simulink model "ModelWithPV"  (R2018a)
settings: Solver=FixedStepAuto  StartTime=0.0  StopTime=1.66  FixedStep=0.01  RelTol=1e-3
PreLoadFcn:
  | myparameterswithpv;
InitFcn:
  | myparameterswithpv;
StopFcn:
  | %datawriter;
values from neighbouring files (symbols this model uses):
  max_p = max(ut_price_i)    [myparametersnopv.m]    (also in myparameterswithpv.m)
libraries: fuzblock x1
settings Model: Creator=timothy  LastModifiedBy=timothy

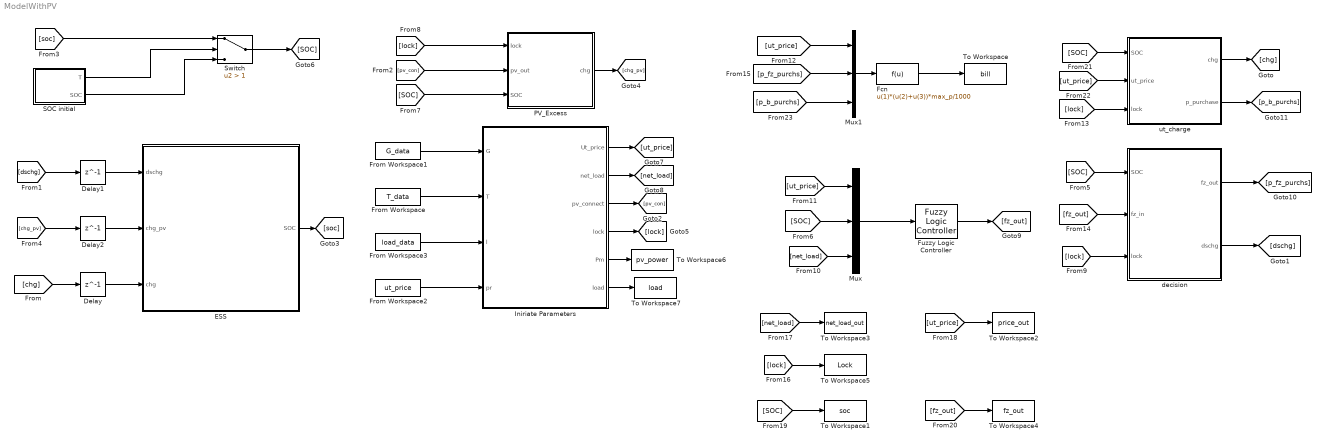
== system ModelWithPV ==
  Delay : Delay  DelayLength=1  InitialCondition=0
  Delay1 : Delay  DelayLength=1  InitialCondition=0
  Delay2 : Delay  DelayLength=1  InitialCondition=0
  ESS : MATLAB Function  TreatAsAtomicUnit=on
  Fcn : Fcn  Expr=u(1)*(u(2)+u(3))*max_p/1000
  From Workspace : FromWorkspace  VariableName=T_data  SampleTime=0
  From Workspace1 : FromWorkspace  VariableName=G_data  SampleTime=0
  From Workspace2 : FromWorkspace  VariableName=ut_price  SampleTime=0
  From Workspace3 : FromWorkspace  VariableName=load_data  SampleTime=0
  Fuzzy Logic Controller : fuzblock/Fuzzy Logic  Controller  FIS=fuzzy_controller  OutputSampleNumber=101  DataType=double  FuzzifiedInputs=off  RuleFiringStrengths=off  RuleOutputs=off  AggregatedOutputs=off  SimulateUsing=Interpreted execution  OutOfRangeInputValueMessage=warning  NoRuleFiredMessage=warning  EmptyOutputFuzzySetMessage=warning
  Iniriate Parameters : MATLAB Function  TreatAsAtomicUnit=on
  Mux : Mux  Inputs=3
  Mux1 : Mux  Inputs=3
  PV_Excess : MATLAB Function  TreatAsAtomicUnit=on
  SOC initial : MATLAB Function  TreatAsAtomicUnit=on
  Switch : Switch  Criteria=u2 > Threshold  Threshold=1
  To Workspace : ToWorkspace  VariableName=bill  SaveFormat=Timeseries  SampleTime=-1
  To Workspace1 : ToWorkspace  VariableName=soc  SaveFormat=Timeseries  SampleTime=-1
  To Workspace2 : ToWorkspace  VariableName=price_out  SaveFormat=Timeseries  SampleTime=-1
  To Workspace3 : ToWorkspace  VariableName=net_load_out  SaveFormat=Timeseries  SampleTime=-1
  To Workspace4 : ToWorkspace  VariableName=fz_out  SaveFormat=Timeseries  SampleTime=-1
  To Workspace5 : ToWorkspace  VariableName=Lock  SaveFormat=Timeseries  SampleTime=-1
  To Workspace6 : ToWorkspace  VariableName=pv_power  SaveFormat=Timeseries  SampleTime=-1
  To Workspace7 : ToWorkspace  VariableName=load  SaveFormat=Timeseries  SampleTime=-1
  decision : MATLAB Function  TreatAsAtomicUnit=on
  ut_charge : MATLAB Function  TreatAsAtomicUnit=on
  wires:
  Mux/1 -> Fuzzy Logic Controller/1
  Fuzzy Logic Controller/1 -> [fz_out]
  Iniriate Parameters/2(net_load) -> [net_load]
  decision/2(dschg) -> [dschg]
  Iniriate Parameters/3(pv_connect) -> [pv_con]
  [pv_con] -> PV_Excess/2(pv_out)
  PV_Excess/1(chg) -> [chg_pv]
  Iniriate Parameters/4(lock) -> [lock]
  ESS/1(SOC) -> [soc]
  [SOC] -> PV_Excess/3(SOC)
  From Workspace3/1 -> Iniriate Parameters/3(l)
  From Workspace/1 -> Iniriate Parameters/2(T)
  From Workspace1/1 -> Iniriate Parameters/1(G)
  From Workspace2/1 -> Iniriate Parameters/4(pr)
  Delay1/1 -> ESS/1(dschg)
  Delay2/1 -> ESS/2(chg_pv)
  [dschg] -> Delay1/1
  [chg_pv] -> Delay2/1
  [soc] -> Switch/1
  SOC initial/1(T) -> Switch/2
  SOC initial/2(SOC) -> Switch/3
  Switch/1 -> [SOC]
  [SOC] -> Mux/2
  decision/1(fz_out) -> [p_fz_purchs]
  Mux1/1 -> Fcn/1
  Fcn/1 -> To Workspace/1
  Iniriate Parameters/1(Ut_price) -> [ut_price]
  [chg] -> Delay/1
  Iniriate Parameters/5(Pm) -> To Workspace6/1
  Delay/1 -> ESS/3(chg)
  [SOC] -> decision/1(SOC)
  [lock] -> PV_Excess/1(lock)
  [lock] -> decision/3(lock)
  [net_load] -> Mux/3
  [ut_price] -> Mux/1
  [ut_price] -> Mux1/1
  [fz_out] -> decision/2(fz_in)
  [p_fz_purchs] -> Mux1/2
  [lock] -> To Workspace5/1
  [net_load] -> To Workspace3/1
  [ut_price] -> To Workspace2/1
  [SOC] -> To Workspace1/1
  [fz_out] -> To Workspace4/1
  ut_charge/1(chg) -> [chg]
  [lock] -> ut_charge/3(lock)
  [SOC] -> ut_charge/1(SOC)
  [ut_price] -> ut_charge/2(ut_price)
  ut_charge/2(p_purchase) -> [p_b_purchs]
  [p_b_purchs] -> Mux1/3
  Iniriate Parameters/6(load) -> To Workspace7/1

== matlab function ModelWithPV/PV_Excess ==
  data: lock input; pv_out input; chg output; SOC input
function chg  = sell_or_charge(lock, pv_out, SOC)

% Decides on whether to charge the battery or sell power
% to the utility
% persistent t;

% if isempty(t) || t == 24
%     t = 1;
% end
% 
% if pv_out(1) > 0 && soc == 100
%     %Sell to the utility
%     chg = 0;
%     sell = 0; % To be determined later
% elseif pv_out(1) > 0 && soc < 100
%     % Charge the battery
%     chg = 2*pv_out(2); %Charging current from the PV
%     sell = 1;
% else
%     %input values set to zeroes
%     chg = 0;
%     sell = 0;
% end
% 
% t = t+1;
if lock == 0
    % Not enough pv output
    chg = 0;
    %sell = 0;
else
    % Excess PV output
    if SOC < 100
        soc_needed = 100 - SOC;
        if 2*pv_out(2) <= soc_needed
            % charge the battery
            chg = 2*pv_out(2);
            %sell = 0;
        else
            % charge the battery and sell the excess
            %sell = 2*pv_out(2)-soc_needed;
            %sell = 1;
            chg = soc_needed;
        end
    else
        % Sell the excess 
        chg = 0;
        %sell = 1;
    end
end

== matlab function ModelWithPV/ESS ==
  data: dschg input; chg_pv input; SOC output; chg input
function SOC = battery(dschg, chg_pv, chg)
% Battery State of charge 
persistent SOC_initial;

%Battery specifications
Q = 340; % Battery capacity in Ah


if isempty(SOC_initial)
    %Initialize the state of charge to 100%
    SOC_initial = 70;
end


% if chg > 0 && chg_pv == 0
%     % Charge the battery
%     SOC = SOC_initial + (100/Q)*chg; %chg is the charging current
% elseif chg == 0 && chg_pv > 0
%     SOC = SOC_initial + (100/Q)*chg_pv; %chg is the charging current
% end
% 
% if dschg > 0 && dschg_pv == 0
%     % Disharge the battery
%     SOC = SOC_initial - (100/Q)*dschg; %dschg is the discharging current
% elseif dschg == 0 && dschg_pv > 0
%     SOC = SOC_initial - (100/Q)*dschg_pv; %dschg_pv is the discharging current
% end

if chg_pv >0
    % PV charging
    SOC = SOC_initial + (100/Q)*chg_pv;
elseif chg > 0
    %Utility charging
    SOC = SOC_initial + (100/Q)*chg;
else
    % Disharge the battery
    SOC = SOC_initial - (100/Q)*dschg;
        
end
SOC_initial = SOC; %Update the battery state of charge

== matlab function ModelWithPV/Iniriate Parameters ==
  data: Ut_price output; net_load output; pv_connect output; lock output; G input; T input; l input; pr input; Pm output; load output
function [Ut_price, net_load, pv_connect, lock, Pm, load] = eval_param(G, T, l, pr)

% Manufacturers data sheet data Solar panel
Pstc = 120;
Cp = 0.45;
Tr = 25;
Gstc = 1000;
Istc = 6.6;
Vstc = 18.1;

persistent t;
%dataType = 'double';

if isempty(t) 
    t = 1;
end

if t == 168
    t = 1;
end
Ut_price = pr(t);
load = l(t);

% Pv output from 4 solar panels
Gi = G(t);
Tm = T(t);
k = Gi/Gstc;
Pmt = Pstc*Cp*abs(Tm-Tr);
Pma = Pstc+Pmt;
if Gi == 0
    Pm = 0;
else
    Pm = 4*(k.*Pma-0.01*Pstc);
end
Imt = k*Istc;

% Net load
net_load_temp = load-Pm;

if net_load_temp > 0
    net_load = net_load_temp;
    pv_connect = [0, 0];
    lock = 0;
else
    pv_connect = [abs(net_load_temp), Imt];
    net_load = 0;
    lock = 1;
end

t = t+1;

== matlab function ModelWithPV/ut_charge ==
  data: SOC input; chg output; ut_price input; lock input; p_purchase output
function [chg, p_purchase] = ut_charge(SOC, ut_price, lock)
% Charges the battery when the Utility prices are low
Q = 340; %Battery capacity
if lock == 1
    %PV power output is enough
    chg = 0;
    p_purchase = 0;
else
    %PV out is less
    %Check the state of charge of the battery
    if SOC >=80
        % No need to charge
        chg = 0;
        p_purchase = 0;
    else
        % Check the utility price
        if ut_price <= 0.3
            %Prices are low for purchasing power
            chg = 0.2*Q; %Charging current limited to 20% of Capacity
            p_purchase = 240*chg; 
        else
            %Prices are high
            chg = 0;
            p_purchase = 0;
        end
    end
end

== matlab function ModelWithPV/SOC initial ==
  data: T output; SOC output
function [T, SOC] = soc_i()

persistent t;
if isempty(t)
    t = 1;
end

if t == 1
    SOC = 100;
else
    SOC = 0;
end
T = t;
t = t+1;

== matlab function ModelWithPV/decision ==
  data: fz_out output; SOC input; fz_in input; dschg output; lock input
function [fz_out, dschg]= decision_intp(SOC, fz_in, lock)
%Q = 340; % Ah
%y = net_load - fz_in;
if lock == 1
    % The output of the pv is in excess and there is no need to run the
    % fuzzy logic controller
    dschg = 0;
    fz_out = 0;
else
    if SOC > 30
       dschg = fz_in/240;
       fz_out = 0;
    else
       dschg = 0;
       fz_out = fz_in;
    end

%     if y > 0 
%         % Connect the battery to compensate
%         % Discharge the battery
%         dschg = y/240; % The discharging current drawn from the battery
%         %chg = 0;
%         fz_out = fz_in;
%         %chg = 0;
%     else
%         % Charge the battery
%         dschg = 0;
%         %chg = abs(y)/240; % The charging current obtained from the utility
%         fz_out = fz_in;
%     end
end
